simulink model "p1_MCU"  (R2023a)
settings: Solver=FixedStepDiscrete  StartTime=0.0  StopTime=inf  FixedStep=Ts_MCU  RelTol=1e-3  EnableMultiTasking=on
PreLoadFcn:
  | p1_params_new
  | spiDataDefinition
InitFcn:
  | mbd_s32k_consistency_checks(bdroot(gcs));
undefined symbols (not defined in the file or in its folder): ack, cpr_handwheel, cpr_steering, Discrete, DriverInput, DrivetrainLeft, DrivetrainRight, LQFP, MPU_IO, n_handwheel, n_steering, p1data, p1params, param, sr, steering_limit, SteeringLeft, SteeringRight, Time, Ts_MCU, wc, WheelForceLeft, WheelForceRight
libraries: simulink x74, mbd_s32k1xx_ec_toolbox x58, Library_Drivetrain x5, Library_Steering x5, etargetslib x3, ctrlSharedLib x1
(part 3 of 4)

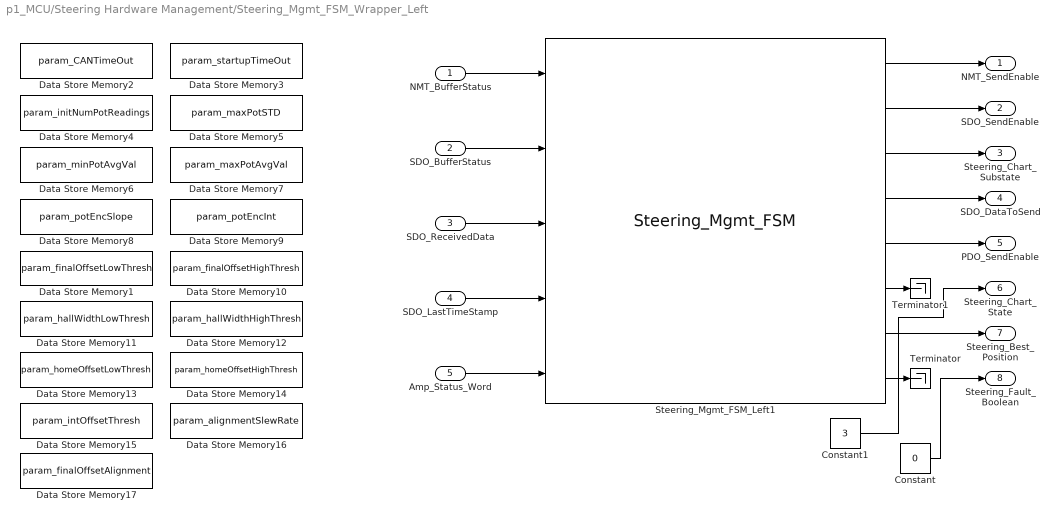
== system p1_MCU/Steering Hardware Management/Steering_Mgmt_FSM_Wrapper_Left ==
  NMT_BufferStatus : Inport
  SDO_BufferStatus : Inport  Port=2
  SDO_ReceivedData : Inport  Port=3
  SDO_LastTimeStamp : Inport  Port=4
  Amp_Status_Word : Inport  Port=5
  Constant : Constant  Value=0  OutDataTypeStr=Inherit: Inherit via back propagation
  Constant1 : Constant  Value=3  OutDataTypeStr=Inherit: Inherit via back propagation
  Data Store Memory1 : DataStoreMemory  DataStoreName=param_finalOffsetLowThresh  ReadBeforeWriteMsg=warning  WriteAfterWriteMsg=warning  WriteAfterReadMsg=warning  InitialValue=p1params.steering.left.finalOffsetLowThresh  ShowAdditionalParam=off  OutDataTypeStr=double
  Data Store Memory10 : DataStoreMemory  DataStoreName=param_finalOffsetHighThresh  ReadBeforeWriteMsg=warning  WriteAfterWriteMsg=warning  WriteAfterReadMsg=warning  InitialValue=p1params.steering.left.finalOffsetHighThresh  ShowAdditionalParam=off  OutDataTypeStr=double
  Data Store Memory11 : DataStoreMemory  DataStoreName=param_hallWidthLowThresh  ReadBeforeWriteMsg=warning  WriteAfterWriteMsg=warning  WriteAfterReadMsg=warning  InitialValue=p1params.steering.left.hallWidthLowThresh  ShowAdditionalParam=off  OutDataTypeStr=double
  Data Store Memory12 : DataStoreMemory  DataStoreName=param_hallWidthHighThresh  ReadBeforeWriteMsg=warning  WriteAfterWriteMsg=warning  WriteAfterReadMsg=warning  InitialValue=p1params.steering.left.hallWidthHighThresh  ShowAdditionalParam=off  OutDataTypeStr=double
  Data Store Memory13 : DataStoreMemory  DataStoreName=param_homeOffsetLowThresh  ReadBeforeWriteMsg=warning  WriteAfterWriteMsg=warning  WriteAfterReadMsg=warning  InitialValue=p1params.steering.left.homeOffsetLowThresh  ShowAdditionalParam=off  OutDataTypeStr=double
  Data Store Memory14 : DataStoreMemory  DataStoreName=param_homeOffsetHighThresh  ReadBeforeWriteMsg=warning  WriteAfterWriteMsg=warning  WriteAfterReadMsg=warning  InitialValue=p1params.steering.left.homeOffsetHighThresh  ShowAdditionalParam=off  OutDataTypeStr=double
  Data Store Memory15 : DataStoreMemory  DataStoreName=param_intOffsetThresh  ReadBeforeWriteMsg=warning  WriteAfterWriteMsg=warning  WriteAfterReadMsg=warning  InitialValue=p1params.steering.left.intOffsetThresh  ShowAdditionalParam=off  OutDataTypeStr=double
  Data Store Memory16 : DataStoreMemory  DataStoreName=param_alignmentSlewRate  ReadBeforeWriteMsg=warning  WriteAfterWriteMsg=warning  WriteAfterReadMsg=warning  InitialValue=p1params.steering.left.alignmentSlewRate  ShowAdditionalParam=off  OutDataTypeStr=double
  Data Store Memory17 : DataStoreMemory  DataStoreName=param_finalOffsetAlignment  ReadBeforeWriteMsg=warning  WriteAfterWriteMsg=warning  WriteAfterReadMsg=warning  InitialValue=p1params.steering.left.finalOffsetAlignment  ShowAdditionalParam=off  OutDataTypeStr=double
  Data Store Memory2 : DataStoreMemory  DataStoreName=param_CANTimeOut  ReadBeforeWriteMsg=warning  WriteAfterWriteMsg=warning  WriteAfterReadMsg=warning  InitialValue=p1params.steering.left.CANTimeOut  ShowAdditionalParam=off  OutDataTypeStr=double
  Data Store Memory3 : DataStoreMemory  DataStoreName=param_startupTimeOut  ReadBeforeWriteMsg=warning  WriteAfterWriteMsg=warning  WriteAfterReadMsg=warning  InitialValue=p1params.steering.left.startupTimeOut  ShowAdditionalParam=off  OutDataTypeStr=double
  Data Store Memory4 : DataStoreMemory  DataStoreName=param_initNumPotReadings  ReadBeforeWriteMsg=warning  WriteAfterWriteMsg=warning  WriteAfterReadMsg=warning  InitialValue=p1params.steering.left.initNumPotReadings  ShowAdditionalParam=off  OutDataTypeStr=double
  Data Store Memory5 : DataStoreMemory  DataStoreName=param_maxPotSTD  ReadBeforeWriteMsg=warning  WriteAfterWriteMsg=warning  WriteAfterReadMsg=warning  InitialValue=p1params.steering.left.maxPotSTD  ShowAdditionalParam=off  OutDataTypeStr=double
  Data Store Memory6 : DataStoreMemory  DataStoreName=param_minPotAvgVal  ReadBeforeWriteMsg=warning  WriteAfterWriteMsg=warning  WriteAfterReadMsg=warning  InitialValue=p1params.steering.left.minPotAvgVal  ShowAdditionalParam=off  OutDataTypeStr=double
  Data Store Memory7 : DataStoreMemory  DataStoreName=param_maxPotAvgVal  ReadBeforeWriteMsg=warning  WriteAfterWriteMsg=warning  WriteAfterReadMsg=warning  InitialValue=p1params.steering.left.maxPotAvgVal  ShowAdditionalParam=off  OutDataTypeStr=double
  Data Store Memory8 : DataStoreMemory  DataStoreName=param_potEncSlope  ReadBeforeWriteMsg=warning  WriteAfterWriteMsg=warning  WriteAfterReadMsg=warning  InitialValue=p1params.steering.left.potEncSlope  ShowAdditionalParam=off  OutDataTypeStr=double
  Data Store Memory9 : DataStoreMemory  DataStoreName=param_potEncInt  ReadBeforeWriteMsg=warning  WriteAfterWriteMsg=warning  WriteAfterReadMsg=warning  InitialValue=p1params.steering.left.potEncInt  ShowAdditionalParam=off  OutDataTypeStr=double
  Steering_Mgmt_FSM_Left1 : Library_Steering/Steering_Mgmt_FSM  SystemSampleTime=-1  VariantActivationTime=update diagram  Latency=0  AutoFrameSizeCalculation=off
  Terminator : Terminator
  Terminator1 : Terminator
  NMT_SendEnable : Outport
  SDO_SendEnable : Outport  Port=2
  Steering_Chart_Substate : Outport  Port=3
  SDO_DataToSend : Outport  Port=4
  PDO_SendEnable : Outport  Port=5
  Steering_Chart_State : Outport  Port=6
  Steering_Best_Position : Outport  Port=7
  Steering_Fault_Boolean : Outport  Port=8
  wires:
  Amp_Status_Word/1 -> Steering_Mgmt_FSM_Left1/5
  Steering_Mgmt_FSM_Left1/2 -> SDO_SendEnable/1
  Steering_Mgmt_FSM_Left1/1 -> NMT_SendEnable/1
  SDO_ReceivedData/1 -> Steering_Mgmt_FSM_Left1/3
  SDO_LastTimeStamp/1 -> Steering_Mgmt_FSM_Left1/4
  SDO_BufferStatus/1 -> Steering_Mgmt_FSM_Left1/2
  NMT_BufferStatus/1 -> Steering_Mgmt_FSM_Left1/1
  Steering_Mgmt_FSM_Left1/8 -> Terminator/1
  Steering_Mgmt_FSM_Left1/7 -> Steering_Best_Position/1
  Steering_Mgmt_FSM_Left1/3 -> Steering_Chart_Substate/1
  Steering_Mgmt_FSM_Left1/4 -> SDO_DataToSend/1
  Steering_Mgmt_FSM_Left1/5 -> PDO_SendEnable/1
  Steering_Mgmt_FSM_Left1/6 -> Terminator1/1
  Constant/1 -> Steering_Fault_Boolean/1
  Constant1/1 -> Steering_Chart_State/1

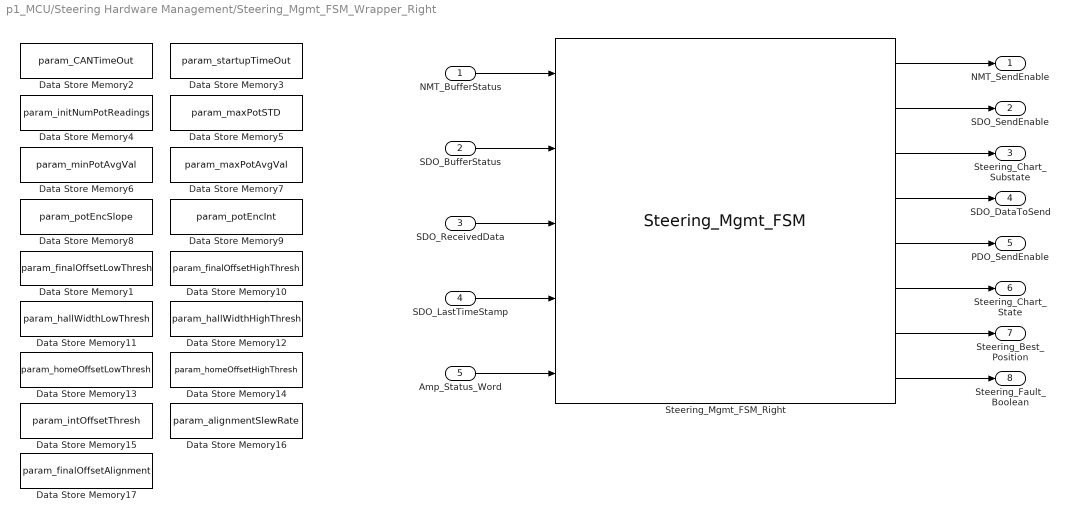
== system p1_MCU/Steering Hardware Management/Steering_Mgmt_FSM_Wrapper_Right ==
  NMT_BufferStatus : Inport
  SDO_BufferStatus : Inport  Port=2
  SDO_ReceivedData : Inport  Port=3
  SDO_LastTimeStamp : Inport  Port=4
  Amp_Status_Word : Inport  Port=5
  Data Store Memory1 : DataStoreMemory  DataStoreName=param_finalOffsetLowThresh  ReadBeforeWriteMsg=warning  WriteAfterWriteMsg=warning  WriteAfterReadMsg=warning  InitialValue=p1params.steering.right.finalOffsetLowThresh  ShowAdditionalParam=off  OutDataTypeStr=double
  Data Store Memory10 : DataStoreMemory  DataStoreName=param_finalOffsetHighThresh  ReadBeforeWriteMsg=warning  WriteAfterWriteMsg=warning  WriteAfterReadMsg=warning  InitialValue=p1params.steering.right.finalOffsetHighThresh  ShowAdditionalParam=off  OutDataTypeStr=double
  Data Store Memory11 : DataStoreMemory  DataStoreName=param_hallWidthLowThresh  ReadBeforeWriteMsg=warning  WriteAfterWriteMsg=warning  WriteAfterReadMsg=warning  InitialValue=p1params.steering.right.hallWidthLowThresh  ShowAdditionalParam=off  OutDataTypeStr=double
  Data Store Memory12 : DataStoreMemory  DataStoreName=param_hallWidthHighThresh  ReadBeforeWriteMsg=warning  WriteAfterWriteMsg=warning  WriteAfterReadMsg=warning  InitialValue=p1params.steering.right.hallWidthHighThresh  ShowAdditionalParam=off  OutDataTypeStr=double
  Data Store Memory13 : DataStoreMemory  DataStoreName=param_homeOffsetLowThresh  ReadBeforeWriteMsg=warning  WriteAfterWriteMsg=warning  WriteAfterReadMsg=warning  InitialValue=p1params.steering.right.homeOffsetLowThresh  ShowAdditionalParam=off  OutDataTypeStr=double
  Data Store Memory14 : DataStoreMemory  DataStoreName=param_homeOffsetHighThresh  ReadBeforeWriteMsg=warning  WriteAfterWriteMsg=warning  WriteAfterReadMsg=warning  InitialValue=p1params.steering.right.homeOffsetHighThresh  ShowAdditionalParam=off  OutDataTypeStr=double
  Data Store Memory15 : DataStoreMemory  DataStoreName=param_intOffsetThresh  ReadBeforeWriteMsg=warning  WriteAfterWriteMsg=warning  WriteAfterReadMsg=warning  InitialValue=p1params.steering.right.intOffsetThresh  ShowAdditionalParam=off  OutDataTypeStr=double
  Data Store Memory16 : DataStoreMemory  DataStoreName=param_alignmentSlewRate  ReadBeforeWriteMsg=warning  WriteAfterWriteMsg=warning  WriteAfterReadMsg=warning  InitialValue=p1params.steering.right.alignmentSlewRate  ShowAdditionalParam=off  OutDataTypeStr=double
  Data Store Memory17 : DataStoreMemory  DataStoreName=param_finalOffsetAlignment  ReadBeforeWriteMsg=warning  WriteAfterWriteMsg=warning  WriteAfterReadMsg=warning  InitialValue=p1params.steering.right.finalOffsetAlignment  ShowAdditionalParam=off  OutDataTypeStr=double
  Data Store Memory2 : DataStoreMemory  DataStoreName=param_CANTimeOut  ReadBeforeWriteMsg=warning  WriteAfterWriteMsg=warning  WriteAfterReadMsg=warning  InitialValue=p1params.steering.right.CANTimeOut  ShowAdditionalParam=off  OutDataTypeStr=double
  Data Store Memory3 : DataStoreMemory  DataStoreName=param_startupTimeOut  ReadBeforeWriteMsg=warning  WriteAfterWriteMsg=warning  WriteAfterReadMsg=warning  InitialValue=p1params.steering.right.startupTimeOut  ShowAdditionalParam=off  OutDataTypeStr=double
  Data Store Memory4 : DataStoreMemory  DataStoreName=param_initNumPotReadings  ReadBeforeWriteMsg=warning  WriteAfterWriteMsg=warning  WriteAfterReadMsg=warning  InitialValue=p1params.steering.right.initNumPotReadings  ShowAdditionalParam=off  OutDataTypeStr=double
  Data Store Memory5 : DataStoreMemory  DataStoreName=param_maxPotSTD  ReadBeforeWriteMsg=warning  WriteAfterWriteMsg=warning  WriteAfterReadMsg=warning  InitialValue=p1params.steering.right.maxPotSTD  ShowAdditionalParam=off  OutDataTypeStr=double
  Data Store Memory6 : DataStoreMemory  DataStoreName=param_minPotAvgVal  ReadBeforeWriteMsg=warning  WriteAfterWriteMsg=warning  WriteAfterReadMsg=warning  InitialValue=p1params.steering.right.minPotAvgVal  ShowAdditionalParam=off  OutDataTypeStr=double
  Data Store Memory7 : DataStoreMemory  DataStoreName=param_maxPotAvgVal  ReadBeforeWriteMsg=warning  WriteAfterWriteMsg=warning  WriteAfterReadMsg=warning  InitialValue=p1params.steering.right.maxPotAvgVal  ShowAdditionalParam=off  OutDataTypeStr=double
  Data Store Memory8 : DataStoreMemory  DataStoreName=param_potEncSlope  ReadBeforeWriteMsg=warning  WriteAfterWriteMsg=warning  WriteAfterReadMsg=warning  InitialValue=p1params.steering.right.potEncSlope  ShowAdditionalParam=off  OutDataTypeStr=double
  Data Store Memory9 : DataStoreMemory  DataStoreName=param_potEncInt  ReadBeforeWriteMsg=warning  WriteAfterWriteMsg=warning  WriteAfterReadMsg=warning  InitialValue=p1params.steering.right.potEncInt  ShowAdditionalParam=off  OutDataTypeStr=double
  Steering_Mgmt_FSM_Right : Library_Steering/Steering_Mgmt_FSM  SystemSampleTime=-1  VariantActivationTime=update diagram  Latency=0  AutoFrameSizeCalculation=off
  NMT_SendEnable : Outport
  SDO_SendEnable : Outport  Port=2
  Steering_Chart_Substate : Outport  Port=3
  SDO_DataToSend : Outport  Port=4
  PDO_SendEnable : Outport  Port=5
  Steering_Chart_State : Outport  Port=6
  Steering_Best_Position : Outport  Port=7
  Steering_Fault_Boolean : Outport  Port=8
  wires:
  Amp_Status_Word/1 -> Steering_Mgmt_FSM_Right/5
  Steering_Mgmt_FSM_Right/2 -> SDO_SendEnable/1
  Steering_Mgmt_FSM_Right/1 -> NMT_SendEnable/1
  SDO_ReceivedData/1 -> Steering_Mgmt_FSM_Right/3
  SDO_LastTimeStamp/1 -> Steering_Mgmt_FSM_Right/4
  SDO_BufferStatus/1 -> Steering_Mgmt_FSM_Right/2
  NMT_BufferStatus/1 -> Steering_Mgmt_FSM_Right/1
  Steering_Mgmt_FSM_Right/8 -> Steering_Fault_Boolean/1
  Steering_Mgmt_FSM_Right/7 -> Steering_Best_Position/1
  Steering_Mgmt_FSM_Right/3 -> Steering_Chart_Substate/1
  Steering_Mgmt_FSM_Right/4 -> SDO_DataToSend/1
  Steering_Mgmt_FSM_Right/5 -> PDO_SendEnable/1
  Steering_Mgmt_FSM_Right/6 -> Steering_Chart_State/1

== system p1_MCU/Subsystem/System Start ==

== system p1_MCU/Subsystem1/piSPISend ==
  Data Store Memory1 : DataStoreMemory  DataStoreName=spiTx  ReadBeforeWriteMsg=warning  WriteAfterWriteMsg=warning  WriteAfterReadMsg=warning  InitialValue=zeros(p1data.spiBytes,1)  ShowAdditionalParam=off  OutDataTypeStr=uint8
  Data Store Memory3 : DataStoreMemory  DataStoreName=spiPadding  ReadBeforeWriteMsg=warning  WriteAfterWriteMsg=warning  WriteAfterReadMsg=warning  InitialValue=zeros(p1data.mcuPadding,1)  ShowAdditionalParam=off  OutDataTypeStr=uint8
  Data Store Read1 : DataStoreRead  DataStoreName=spiTx  IndexOptions=Index vector (dialog)  Indices=1  OutputSizes=1
  Data Store Read10 : DataStoreRead  DataStoreName=WheelForceRight  IndexOptions=Index vector (dialog)  Indices=1  OutputSizes=1
  Data Store Read11 : DataStoreRead  DataStoreName=spiRx  IndexOptions=Index vector (dialog)  Indices=1  OutputSizes=1
  Data Store Read12 : DataStoreRead  DataStoreName=IMU  IndexOptions=Index vector (dialog)  Indices=1  OutputSizes=1
  Data Store Read14 : DataStoreRead  DataStoreName=spiPadding  IndexOptions=Index vector (dialog)  Indices=1  OutputSizes=1
  Data Store Read2 : DataStoreRead  DataStoreName=IgnState  IndexOptions=Index vector (dialog)  Indices=1  OutputSizes=1
  Data Store Read3 : DataStoreRead  DataStoreName=ControlPanel  IndexOptions=Index vector (dialog)  Indices=1  OutputSizes=1
  Data Store Read4 : DataStoreRead  DataStoreName=SteeringRight  IndexOptions=Index vector (dialog)  Indices=1  OutputSizes=1
  Data Store Read5 : DataStoreRead  DataStoreName=DriverInput  IndexOptions=Index vector (dialog)  Indices=1  OutputSizes=1
  Data Store Read6 : DataStoreRead  DataStoreName=SteeringLeft  IndexOptions=Index vector (dialog)  Indices=1  OutputSizes=1
  Data Store Read7 : DataStoreRead  DataStoreName=DrivetrainLeft  IndexOptions=Index vector (dialog)  Indices=1  OutputSizes=1
  Data Store Read8 : DataStoreRead  DataStoreName=DrivetrainRight  IndexOptions=Index vector (dialog)  Indices=1  OutputSizes=1
  Data Store Read9 : DataStoreRead  DataStoreName=WheelForceLeft  IndexOptions=Index vector (dialog)  Indices=1  OutputSizes=1
  Data Store Write1 : DataStoreWrite  DataStoreName=spiTx  IndexOptions=Index vector (dialog)  Indices=1  OutputSizes=1
  Data Store Write2 : DataStoreWrite  DataStoreName=spiRx  IndexOptions=Index vector (dialog)  Indices=1  OutputSizes=1
  Data Store Write3 : DataStoreWrite  DataStoreName=MPU_IO  IndexOptions=Index vector (dialog)  Indices=1  OutputSizes=1
  Data Store Write5 : DataStoreWrite  DataStoreName=GPS  IndexOptions=Index vector (dialog)  Indices=1  OutputSizes=1
  Demux : Demux  Outputs=3
  Footer : Constant  Value=[0 0 101 110 100]  OutDataTypeStr=uint8
  Header : Constant  Value=[115 116 97 114 116 0 0 0 0 0]  OutDataTypeStr=uint8
  LPSPI_Slave_Transfer : mbd_s32k1xx_ec_toolbox/Communication Blocks/SPI Blocks/LPSPI_Slave_Transfer  instance=1  pcs=3  pcs_polarity=ActiveLow  xfermode=Non blocking  timeout=70  spi_upd=on
  Mux1 : Mux  Inputs=13
  Terminator : Terminator
  wires:
  Data Store Read8/1 -> Mux1/8
  Data Store Read2/1 -> Mux1/2
  Data Store Read4/1 -> Mux1/6
  Mux1/1 -> Data Store Write1/1
  LPSPI_Slave_Transfer/1 -> Data Store Write2/1
  Data Store Read1/1 -> LPSPI_Slave_Transfer/1
  Data Store Read11/1 -> Demux/1
  Data Store Read6/1 -> Mux1/5
  Data Store Read7/1 -> Mux1/7
  Data Store Read5/1 -> Mux1/4
  Data Store Read3/1 -> Mux1/3
  Demux/3 -> Terminator/1
  Demux/1 -> Data Store Write5/1
  Demux/2 -> Data Store Write3/1
  Data Store Read10/1 -> Mux1/11
  Data Store Read9/1 -> Mux1/10
  Data Store Read12/1 -> Mux1/9
  Header/1 -> Mux1/1
  Data Store Read14/1 -> Mux1/12
  Footer/1 -> Mux1/13

== system p1_MCU/Subsystem2/If Action Subsystem ==
  note: Start interrupt-based reception
      | on CAN1 bus
  note: Enable CAN1 bus
  note: Hold Power On (Ignition)
  note: Enable 5V Output
  note: Enable CAN0 bus
  note: Start interrupt-based reception
      | on CAN0 bus
  note: Enable CAN2 bus
  note: Enable Digital Outputs
  note: Enable Digital Input Pullups
  Action Port : ActionPort  ActionPortLabel=if(u1 == 0)
  Constant : Constant  OutDataTypeStr=uint32
  Constant{1..2,5..6} (4 alike) : Constant  OutDataTypeStr=Inherit: Inherit via back propagation
  Constant3 : Constant  Value=0  OutDataTypeStr=Inherit: Inherit via back propagation
  Constant4 : Constant  Value=0  OutDataTypeStr=Inherit: Inherit via back propagation
  Constant9 : Constant  Value=0  OutDataTypeStr=Inherit: Inherit via back propagation
  Digital_Output : mbd_s32k1xx_ec_toolbox/GPIO Blocks/Digital_Output  gpio_pin=PTA14: [PTA14 | Port A I/O]  init_val=Low  drive_strength=Low
  Digital_Output1 : mbd_s32k1xx_ec_toolbox/GPIO Blocks/Digital_Output  gpio_pin=PTE7: [PTE7 | Port E I/O]  init_val=Low  drive_strength=Low
  Digital_Output2 : mbd_s32k1xx_ec_toolbox/GPIO Blocks/Digital_Output  gpio_pin=PTD7: [PTD7 | Port D I/O]  init_val=High  drive_strength=Low
  Digital_Output3 : mbd_s32k1xx_ec_toolbox/GPIO Blocks/Digital_Output  gpio_pin=PTC10: [PTC10 | Port C I/O]  init_val=Low  drive_strength=Low
  Digital_Output4 : mbd_s32k1xx_ec_toolbox/GPIO Blocks/Digital_Output  gpio_pin=PTD6: [PTD6 | Port D I/O]  init_val=Low  drive_strength=Low
  Digital_Output5 : mbd_s32k1xx_ec_toolbox/GPIO Blocks/Digital_Output  gpio_pin=PTE3: [PTE3 | Port E I/O]  init_val=Low  drive_strength=Low
  Digital_Output6 : mbd_s32k1xx_ec_toolbox/GPIO Blocks/Digital_Output  gpio_pin=PTC8: [PTC8 | Port C I/O]  init_val=Low  drive_strength=Low
  Enable_Handwheel_Index_Capture_Once : mbd_s32k1xx_ec_toolbox/GPIO Blocks/Digital_Input_ISR_Enable_Disable  gpio_pin=PTD10: [PTD10 | Port D I/O]  irqc=on either-edge
  FCAN_Receive : mbd_s32k1xx_ec_toolbox/Communication Blocks/CAN Blocks/FCAN_Receive  can_instance=1  can_mode=Non-blocking  can_timeout_ms=0  can_mb_idx=0  can_extended_id=off  can_is_remote=off  can_id=0  can_msg_mask=0  show_adv_opts=off  can_use_rxfifo=off  can_fd_enable=off
  FCAN_Receive1 : mbd_s32k1xx_ec_toolbox/Communication Blocks/CAN Blocks/FCAN_Receive  can_instance=0  can_mode=Non-blocking  can_timeout_ms=0  can_mb_idx=0  can_extended_id=off  can_is_remote=off  can_id=0  can_msg_mask=0  show_adv_opts=off  can_use_rxfifo=off  can_fd_enable=off
  FCAN_Receive2 : mbd_s32k1xx_ec_toolbox/Communication Blocks/CAN Blocks/FCAN_Receive  can_instance=2  can_mode=Non-blocking  can_timeout_ms=0  can_mb_idx=7  can_extended_id=off  can_is_remote=off  can_id=0  can_msg_mask=0  show_adv_opts=off  can_use_rxfifo=off  can_fd_enable=off
  IMU Reception : Subsystem
  Init Flag Write : DataStoreWrite  DataStoreName=init_flag  IndexOptions=Index vector (dialog)  Indices=1  OutputSizes=1
  wires:
  Constant/1 -> Init Flag Write/1
  Constant9/1 -> Digital_Output/1
  Constant2/1 -> Digital_Output2/1
  Constant1/1 -> Digital_Output1/1
  Constant3/1 -> Digital_Output3/1
  Constant4/1 -> Digital_Output4/1
  Constant5/1 -> Digital_Output5/1
  Constant6/1 -> Digital_Output6/1

== system p1_MCU/WFT CAN Receive/Function-Call Subsystem ==
  Message Buffer : Inport
  MSG ID : Inport  Port=2
  Data Packet : Inport  Port=3
  Data Length : Inport  Port=4
  Time Stamp : Inport  Port=5
  function : TriggerPort  TriggerType=function-call  VariantControl=Variant
  Accurate Feedback2 : Subsystem  TreatAsAtomicUnit=on
      settings: RTWSystemCode=Inline
  Accurate Feedback3 : Subsystem  TreatAsAtomicUnit=on
      settings: RTWSystemCode=Inline
  Bus Creator : BusCreator  Inputs=10
  Bus Creator1 : BusCreator  Inputs=10
  Data Store Write1 : DataStoreWrite  DataStoreName=WheelForceLeft  DataStoreElements=WheelForceLeft(1:8)  IndexOptions=Index vector (dialog)  Indices=1  OutputSizes=1
  Data Store Write2 : DataStoreWrite  DataStoreName=WheelForceLeft  DataStoreElements=WheelForceLeft(9:16)  IndexOptions=Index vector (dialog)  Indices=1  OutputSizes=1
  Data Store Write3 : DataStoreWrite  DataStoreName=WheelForceRight  DataStoreElements=WheelForceRight(1:8)  IndexOptions=Index vector (dialog)  Indices=1  OutputSizes=1
  Data Store Write4 : DataStoreWrite  DataStoreName=WheelForceRight  DataStoreElements=WheelForceRight(9:16)  IndexOptions=Index vector (dialog)  Indices=1  OutputSizes=1
  Data Store Write5 : DataStoreWrite  DataStoreName=WheelForceLeft  DataStoreElements=WheelForceLeft(17:20)  IndexOptions=Index vector (dialog)  Indices=1  OutputSizes=1
  Data Store Write6 : DataStoreWrite  DataStoreName=WheelForceRight  DataStoreElements=WheelForceRight(17:20)  IndexOptions=Index vector (dialog)  Indices=1  OutputSizes=1
  FCAN_Receive : mbd_s32k1xx_ec_toolbox/Communication Blocks/CAN Blocks/FCAN_Receive  can_instance=2  can_mode=Non-blocking  can_timeout_ms=0  can_mb_idx=7  can_extended_id=off  can_is_remote=off  can_id=0  can_msg_mask=0  show_adv_opts=off  can_use_rxfifo=off  can_fd_enable=off
  Switch Case : SwitchCase  CaseConditions={hex2dec('1CC'),hex2dec('5CC'),hex2dec('3CC'),hex2dec('1C7'),hex2dec('5C7'),hex2dec('3C7')}  ShowDefaultCase=off
  Terminator : Terminator
  Terminator1 : Terminator
  Terminator2 : Terminator
  WFT Packet 1 Left : Subsystem  TreatAsAtomicUnit=on
      settings: RTWSystemCode=Inline
  WFT Packet 1 Left1 : Subsystem  TreatAsAtomicUnit=on
      settings: RTWSystemCode=Inline
  WFT Packet 1 Left2 : Subsystem  TreatAsAtomicUnit=on
      settings: RTWSystemCode=Inline
  WFT Packet 1 Left3 : Subsystem  TreatAsAtomicUnit=on
      settings: RTWSystemCode=Inline
  WFT Feedback Left : Outport
  WFT Feedback Right : Outport  Port=2
  wires:
  WFT Packet 1 Left/2(Fx) -> Bus Creator/1  "Fx Left"
  WFT Packet 1 Left/1(Save Data) -> Data Store Write1/1
  WFT Packet 1 Left/4(Fz) -> Bus Creator/3  "Fz Left"
  Switch Case/1 -> WFT Packet 1 Left/Action
  WFT Packet 1 Left/5(Mx) -> Bus Creator/4  "Mx Left"
  Data Length/1 -> Terminator/1
  Bus Creator/1 -> WFT Feedback Left/1
  Message Buffer/1 -> Terminator1/1
  MSG ID/1 -> Switch Case/1
  WFT Packet 1 Left/3(Fy) -> Bus Creator/2  "Fy Left"
  Data Packet/1 -> WFT Packet 1 Left3/1(Data Packet), Accurate Feedback3/1(Data Packet), Accurate Feedback2/1(Data Packet), WFT Packet 1 Left2/1(Data Packet), WFT Packet 1 Left1/1(Data Packet), WFT Packet 1 Left/1(Data Packet)
  WFT Packet 1 Left1/1(Save Data) -> Data Store Write2/1
  WFT Packet 1 Left1/5(Pos) -> Bus Creator/8  "Pos Left"
  WFT Packet 1 Left1/3(Mz) -> Bus Creator/6  "Mz Left"
  WFT Packet 1 Left1/4(Vel) -> Bus Creator/7  "Vel Left"
  Switch Case/2 -> WFT Packet 1 Left1/Action
  WFT Packet 1 Left1/2(My) -> Bus Creator/5  "My Left"
  Accurate Feedback2/1(Save Data) -> Data Store Write3/1
  Switch Case/5 -> Accurate Feedback3/Action
  Accurate Feedback3/1(Save Data) -> Data Store Write4/1
  Switch Case/4 -> Accurate Feedback2/Action
  WFT Packet 1 Left2/2(Ax) -> Bus Creator/9  "Ax Left"
  Switch Case/3 -> WFT Packet 1 Left2/Action
  WFT Packet 1 Left2/3(Az) -> Bus Creator/10  "Ay Left"
  WFT Packet 1 Left2/1(Save Data) -> Data Store Write5/1
  Switch Case/6 -> WFT Packet 1 Left3/Action
  Accurate Feedback3/4(Vel) -> Bus Creator1/7  "Vel Right"
  Accurate Feedback3/2(My) -> Bus Creator1/5  "My Right"
  Accurate Feedback2/5(Mx) -> Bus Creator1/4  "Mx Right"
  Accurate Feedback2/3(Fy) -> Bus Creator1/2  "Fy Right"
  WFT Packet 1 Left3/3(Az) -> Bus Creator1/10  "Ay Right"
  Bus Creator1/1 -> WFT Feedback Right/1
  Accurate Feedback2/2(Fx) -> Bus Creator1/1  "Fx Right"
  WFT Packet 1 Left3/2(Ax) -> Bus Creator1/9  "Ax Right"
  Accurate Feedback3/3(Mz) -> Bus Creator1/6  "Mz Right"
  Accurate Feedback3/5(Pos) -> Bus Creator1/8  "Pos Right"
  Accurate Feedback2/4(Fz) -> Bus Creator1/3  "Fz Right"
  WFT Packet 1 Left3/1(Save Data) -> Data Store Write6/1
  Time Stamp/1 -> Terminator2/1

== system p1_MCU/ Controls Data Reception/Function-Call Subsystem1/If Action Subsystem ==
  Raw Encoder Estimate : Inport
  Fused Angle Estimate : Inport  Port=2
  SimTime : Inport  Port=3
  Action Port : ActionPort  ActionPortLabel=if(u1 > 0.1)
  1-D Lookup Table : Lookup_n-D  NumberOfTableDimensions=1  BreakpointsForDimension1=pi/180*[-7.2*30:7.2:30*7.2]  Table=pi/180*[-7.2*30:7.2:30*7.2]  InterpMethod=Nearest  InternalRulePriority=Speed  RndMeth=Simplest
  Digital_Input_ISR_Enable_Disable : mbd_s32k1xx_ec_toolbox/GPIO Blocks/Digital_Input_ISR_Enable_Disable  gpio_pin=PTD10: [PTD10 | Port D I/O]  irqc=request disabled
  Subtract : Sum  Inputs=-+
  Latched Encoder Offset : Outport  InitialOutput=[0]
  Time of Latch : Outport  Port=2  InitialOutput=[0]
  wires:
  Subtract/1 -> Latched Encoder Offset/1
  Fused Angle Estimate/1 -> 1-D Lookup Table/1
  Raw Encoder Estimate/1 -> Subtract/2
  1-D Lookup Table/1 -> Subtract/1
  SimTime/1 -> Time of Latch/1

== system p1_MCU/Steering Control/Steering Controller/Ackermann Correction ==
  Ackermann Angle : Inport
  left ackermann ideal correction angle : Fcn  Expr=u/(1-u*ack*param.d/2/(param.a+param.b))
  right ackermann ideal correction angle : Fcn  Expr=u/(1+u*ack*param.d/2/(param.a+param.b))
  L Steer Angle : Outport
  R Steer Angle : Outport  Port=2
  wires:
  Ackermann Angle/1 -> right ackermann ideal correction angle/1, left ackermann ideal correction angle/1
  right ackermann ideal correction angle/1 -> R Steer Angle/1
  left ackermann ideal correction angle/1 -> L Steer Angle/1

== system p1_MCU/Steering Control/Steering Controller/HAL-9000 ==
  Trigger : Inport
  Amplitude : Constant  Value=amplitude*sr*pi/180
  Chirp Signal : Subsystem  mask(chirp){f1=startfreq, T=duration, f2=endfreq, VectorParams1D=on}
      mask prompts: f1 "Initial frequency (Hz):"; T "Target time (secs):"; f2 "Frequency at target time (Hz):"; VectorParams1D "Interpret vectors parameters as 1-D"
      mask help: Output a linear chirp signal (sine wave whose frequency varies linearly with time).
      mask init:
      | blkName = gcb;
      | t=[0:.1:5];
      | set_param([blkName '/targetTime'], 'VectorParams1D', VectorParams1D);
      | set_param([blkName '/initialFreq'], 'VectorParams1D', VectorParams1D);
      | set_param([blkName '/deltaFreq'], 'VectorParams1D', VectorParams1D);
      mask Help: The chirp signal has linearly increasing frequency with time.  This block can be used for spectral analysis of nonlinear systems.
      mask Display: plot(t,sin(t.*t))
  Constant : Constant
  Constant1 : Constant  Value=0
  Delay : Constant  Value=delay
  Digital Clock : DigitalClock  SampleTime=Ts_MCU
  Double chirp : Subsystem
  Double-step : Subsystem
      mask Display: plot([0 1 1 2 2 3 3 4 4 5],[0 0 1 1 0 0 -1 -1 0 0])
  Enable : Constant  Value=enabled
  Latch : Subsystem  TreatAsAtomicUnit=on
  Maneuver : Constant  Value=maneuver
  Multiport Switch : MultiPortSwitch  Inputs=5  SaturateOnIntegerOverflow=off  InputSameDT=off
  Product : Product  Inputs=3  SaturateOnIntegerOverflow=on  OutDataTypeStr=Inherit: Same as first input
  Product1 : Product  SaturateOnIntegerOverflow=on  OutDataTypeStr=Inherit: Same as first input
  Ramp : Subsystem
      mask Display: plot([0 3 7 10],[1 1 8 8])
  Step : Subsystem
      mask Display: plot([0 5 5 10],[1 1 8 8])
  Sum : Sum  Inputs=|++
  Switch : Switch  Criteria=u2 ~= 0  SaturateOnIntegerOverflow=off  InputSameDT=off
  Offset : Outport
  wires:
  Double chirp/1(Out1) -> Multiport Switch/6
  Double-step/1(Out) -> Multiport Switch/5
  Enable/1 -> Product1/2
  Trigger/1 -> Switch/2
  Delay/1 -> Sum/2
  Latch/1(Out1) -> Sum/1
  Chirp Signal/1(Out2) -> Multiport Switch/4
  Ramp/1(Out1) -> Multiport Switch/3
  Sum/1 -> Double chirp/1(In1), Double-step/1(Start Time), Chirp Signal/1(Start Time), Ramp/1(Start Time), Step/1(Start Time)
  Maneuver/1 -> Multiport Switch/1
  Step/1(Out) -> Multiport Switch/2
  Amplitude/1 -> Product/3
  Multiport Switch/1 -> Product/2
  Product/1 -> Offset/1
  Product1/1 -> Latch/Trigger, Product/1
  Digital Clock/1 -> Latch/1(In1)
  Switch/1 -> Product1/1
  Constant1/1 -> Switch/3
  Constant/1 -> Switch/1

== system p1_MCU/Subsystem2/If Action Subsystem/IMU Reception ==
  Constant1 : Constant  Value=[hex2dec('10'); hex2dec('50'); hex2dec('50')]  OutDataTypeStr=uint8
  LPSPI_Master_Transfer : mbd_s32k1xx_ec_toolbox/Communication Blocks/SPI Blocks/LPSPI_Master_Transfer  instance=0  pcs=2  pcs_polarity=ActiveLow  xfermode=Non blocking  timeout=50  spi_upd=on
  Terminator : Terminator
  wires:
  Constant1/1 -> LPSPI_Master_Transfer/1
  LPSPI_Master_Transfer/1 -> Terminator/1

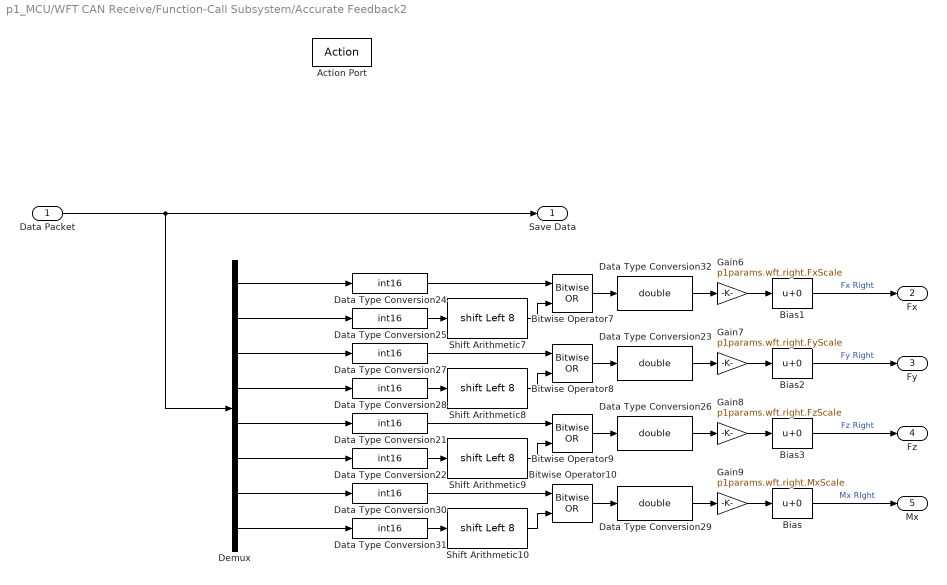
== system p1_MCU/WFT CAN Receive/Function-Call Subsystem/Accurate Feedback2 ==
  Data Packet : Inport
  Action Port : ActionPort  ActionPortLabel=case [ 455 ]:
  Bias{,1..3} (4 alike) : Bias  SaturateOnIntegerOverflow=off
  Bitwise Operator{7..10} (4 alike) : simulink/Logic and Bit Operations/Bitwise Operator  logicop=OR  UseBitMask=off  NumInputPorts=2  BitMask=bin2dec('11011001')  BitMaskRealWorld=Stored Integer
  Data Type Conversion{21..22,24..25,27..28,30..31} (8 alike) : DataTypeConversion  OutDataTypeStr=int16  SaturateOnIntegerOverflow=off  RndMeth=Floor
  Data Type Conversion{23,26,29,32} (4 alike) : DataTypeConversion  OutDataTypeStr=double  SaturateOnIntegerOverflow=off  RndMeth=Floor
  Demux : Demux  Outputs=8
  Gain6 : Gain  Gain=p1params.wft.right.FxScale  OutDataTypeStr=Inherit: Inherit via back propagation
  Gain7 : Gain  Gain=p1params.wft.right.FyScale  OutDataTypeStr=Inherit: Inherit via back propagation
  Gain8 : Gain  Gain=p1params.wft.right.FzScale  OutDataTypeStr=Inherit: Inherit via back propagation
  Gain9 : Gain  Gain=p1params.wft.right.MxScale  OutDataTypeStr=Inherit: Inherit via back propagation
  Shift Arithmetic{7..10} (4 alike) : ArithShift  BitShiftNumber=8  BitShiftDirection=Left
  Save Data : Outport
  Fx : Outport  Port=2
  Fy : Outport  Port=3
  Fz : Outport  Port=4
  Mx : Outport  Port=5
  wires:
  Data Packet/1 -> Save Data/1, Demux/1
  Demux/8 -> Data Type Conversion31/1
  Demux/7 -> Data Type Conversion30/1
  Demux/6 -> Data Type Conversion22/1
  Demux/5 -> Data Type Conversion21/1
  Demux/4 -> Data Type Conversion28/1
  Demux/3 -> Data Type Conversion27/1
  Demux/2 -> Data Type Conversion25/1
  Demux/1 -> Data Type Conversion24/1
  Data Type Conversion23/1 -> Gain7/1
  Shift Arithmetic9/1 -> Bitwise Operator9/2
  Shift Arithmetic8/1 -> Bitwise Operator8/2
  Data Type Conversion25/1 -> Shift Arithmetic7/1
  Data Type Conversion31/1 -> Shift Arithmetic10/1
  Bitwise Operator7/1 -> Data Type Conversion32/1
  Data Type Conversion29/1 -> Gain9/1
  Data Type Conversion27/1 -> Bitwise Operator8/1
  Shift Arithmetic10/1 -> Bitwise Operator10/2
  Gain6/1 -> Bias1/1
  Bitwise Operator8/1 -> Data Type Conversion23/1
  Bitwise Operator10/1 -> Data Type Conversion29/1
  Data Type Conversion26/1 -> Gain8/1
  Gain8/1 -> Bias3/1
  Shift Arithmetic7/1 -> Bitwise Operator7/2
  Data Type Conversion32/1 -> Gain6/1
  Data Type Conversion28/1 -> Shift Arithmetic8/1
  Gain9/1 -> Bias/1
  Bitwise Operator9/1 -> Data Type Conversion26/1
  Data Type Conversion21/1 -> Bitwise Operator9/1
  Data Type Conversion22/1 -> Shift Arithmetic9/1
  Data Type Conversion30/1 -> Bitwise Operator10/1
  Gain7/1 -> Bias2/1
  Data Type Conversion24/1 -> Bitwise Operator7/1
  Bias/1 -> Mx/1  "Mx RIght"
  Bias3/1 -> Fz/1  "Fz Right"
  Bias2/1 -> Fy/1  "Fy Right"
  Bias1/1 -> Fx/1  "Fx Right"

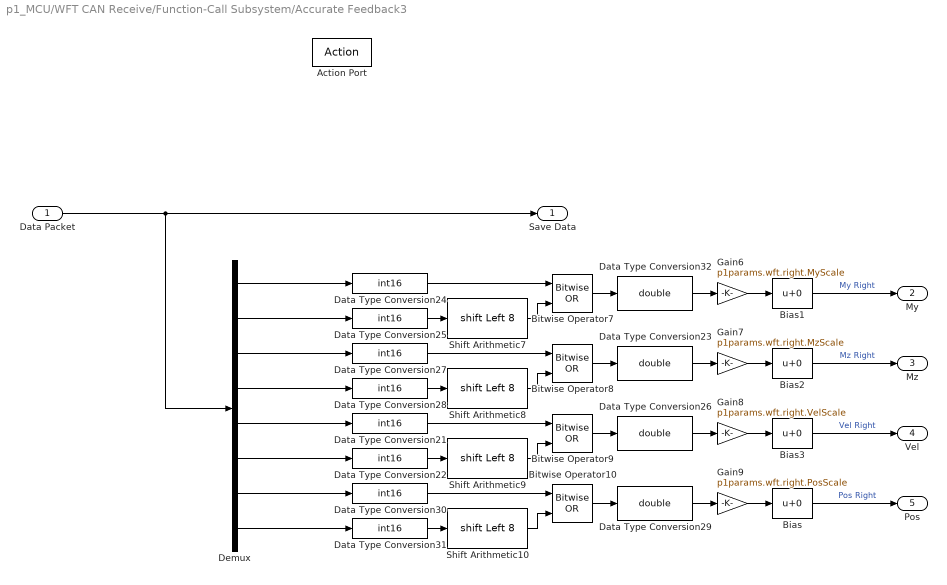
== system p1_MCU/WFT CAN Receive/Function-Call Subsystem/Accurate Feedback3 ==
  Data Packet : Inport
  Action Port : ActionPort  ActionPortLabel=case [ 1479 ]:
  Bias{,1..3} (4 alike) : Bias  SaturateOnIntegerOverflow=off
  Bitwise Operator{7..10} (4 alike) : simulink/Logic and Bit Operations/Bitwise Operator  logicop=OR  UseBitMask=off  NumInputPorts=2  BitMask=bin2dec('11011001')  BitMaskRealWorld=Stored Integer
  Data Type Conversion{21..22,24..25,27..28,30..31} (8 alike) : DataTypeConversion  OutDataTypeStr=int16  SaturateOnIntegerOverflow=off  RndMeth=Floor
  Data Type Conversion{23,26,29,32} (4 alike) : DataTypeConversion  OutDataTypeStr=double  SaturateOnIntegerOverflow=off  RndMeth=Floor
  Demux : Demux  Outputs=8
  Gain6 : Gain  Gain=p1params.wft.right.MyScale  OutDataTypeStr=Inherit: Inherit via back propagation
  Gain7 : Gain  Gain=p1params.wft.right.MzScale  OutDataTypeStr=Inherit: Inherit via back propagation
  Gain8 : Gain  Gain=p1params.wft.right.VelScale  OutDataTypeStr=Inherit: Inherit via back propagation
  Gain9 : Gain  Gain=p1params.wft.right.PosScale  OutDataTypeStr=Inherit: Inherit via back propagation
  Shift Arithmetic{7..10} (4 alike) : ArithShift  BitShiftNumber=8  BitShiftDirection=Left
  Save Data : Outport
  My : Outport  Port=2
  Mz : Outport  Port=3
  Vel : Outport  Port=4
  Pos : Outport  Port=5
  wires:
  Data Packet/1 -> Save Data/1, Demux/1
  Demux/8 -> Data Type Conversion31/1
  Demux/7 -> Data Type Conversion30/1
  Demux/6 -> Data Type Conversion22/1
  Demux/5 -> Data Type Conversion21/1
  Demux/4 -> Data Type Conversion28/1
  Demux/3 -> Data Type Conversion27/1
  Demux/2 -> Data Type Conversion25/1
  Demux/1 -> Data Type Conversion24/1
  Data Type Conversion23/1 -> Gain7/1
  Shift Arithmetic9/1 -> Bitwise Operator9/2
  Shift Arithmetic8/1 -> Bitwise Operator8/2
  Data Type Conversion25/1 -> Shift Arithmetic7/1
  Data Type Conversion31/1 -> Shift Arithmetic10/1
  Bitwise Operator7/1 -> Data Type Conversion32/1
  Data Type Conversion29/1 -> Gain9/1
  Data Type Conversion27/1 -> Bitwise Operator8/1
  Shift Arithmetic10/1 -> Bitwise Operator10/2
  Gain6/1 -> Bias1/1
  Bitwise Operator8/1 -> Data Type Conversion23/1
  Bitwise Operator10/1 -> Data Type Conversion29/1
  Data Type Conversion26/1 -> Gain8/1
  Gain8/1 -> Bias3/1
  Shift Arithmetic7/1 -> Bitwise Operator7/2
  Data Type Conversion32/1 -> Gain6/1
  Data Type Conversion28/1 -> Shift Arithmetic8/1
  Gain9/1 -> Bias/1
  Bitwise Operator9/1 -> Data Type Conversion26/1
  Data Type Conversion21/1 -> Bitwise Operator9/1
  Data Type Conversion22/1 -> Shift Arithmetic9/1
  Data Type Conversion30/1 -> Bitwise Operator10/1
  Gain7/1 -> Bias2/1
  Data Type Conversion24/1 -> Bitwise Operator7/1
  Bias/1 -> Pos/1  "Pos Right"
  Bias3/1 -> Vel/1  "Vel Right"
  Bias2/1 -> Mz/1  "Mz Right"
  Bias1/1 -> My/1  "My Right"

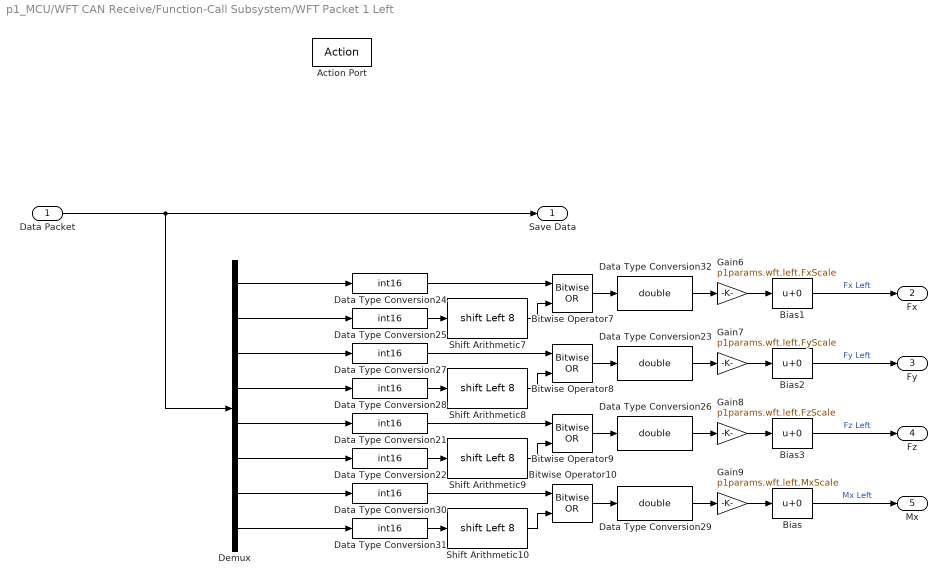
== system p1_MCU/WFT CAN Receive/Function-Call Subsystem/WFT Packet 1 Left ==
  Data Packet : Inport
  Action Port : ActionPort  ActionPortLabel=case [ 460 ]:
  Bias{,1..3} (4 alike) : Bias  SaturateOnIntegerOverflow=off
  Bitwise Operator{7..10} (4 alike) : simulink/Logic and Bit Operations/Bitwise Operator  logicop=OR  UseBitMask=off  NumInputPorts=2  BitMask=bin2dec('11011001')  BitMaskRealWorld=Stored Integer
  Data Type Conversion{21..22,24..25,27..28,30..31} (8 alike) : DataTypeConversion  OutDataTypeStr=int16  SaturateOnIntegerOverflow=off  RndMeth=Floor
  Data Type Conversion{23,26,29,32} (4 alike) : DataTypeConversion  OutDataTypeStr=double  SaturateOnIntegerOverflow=off  RndMeth=Floor
  Demux : Demux  Outputs=8
  Gain6 : Gain  Gain=p1params.wft.left.FxScale  OutDataTypeStr=Inherit: Inherit via back propagation
  Gain7 : Gain  Gain=p1params.wft.left.FyScale  OutDataTypeStr=Inherit: Inherit via back propagation
  Gain8 : Gain  Gain=p1params.wft.left.FzScale  OutDataTypeStr=Inherit: Inherit via back propagation
  Gain9 : Gain  Gain=p1params.wft.left.MxScale  OutDataTypeStr=Inherit: Inherit via back propagation
  Shift Arithmetic{7..10} (4 alike) : ArithShift  BitShiftNumber=8  BitShiftDirection=Left
  Save Data : Outport
  Fx : Outport  Port=2
  Fy : Outport  Port=3
  Fz : Outport  Port=4
  Mx : Outport  Port=5
  wires:
  Data Packet/1 -> Save Data/1, Demux/1
  Demux/8 -> Data Type Conversion31/1
  Demux/7 -> Data Type Conversion30/1
  Demux/6 -> Data Type Conversion22/1
  Demux/5 -> Data Type Conversion21/1
  Demux/4 -> Data Type Conversion28/1
  Demux/3 -> Data Type Conversion27/1
  Demux/2 -> Data Type Conversion25/1
  Demux/1 -> Data Type Conversion24/1
  Data Type Conversion23/1 -> Gain7/1
  Shift Arithmetic9/1 -> Bitwise Operator9/2
  Shift Arithmetic8/1 -> Bitwise Operator8/2
  Data Type Conversion25/1 -> Shift Arithmetic7/1
  Data Type Conversion31/1 -> Shift Arithmetic10/1
  Bitwise Operator7/1 -> Data Type Conversion32/1
  Data Type Conversion29/1 -> Gain9/1
  Data Type Conversion27/1 -> Bitwise Operator8/1
  Shift Arithmetic10/1 -> Bitwise Operator10/2
  Gain6/1 -> Bias1/1
  Bitwise Operator8/1 -> Data Type Conversion23/1
  Bitwise Operator10/1 -> Data Type Conversion29/1
  Data Type Conversion26/1 -> Gain8/1
  Gain8/1 -> Bias3/1
  Shift Arithmetic7/1 -> Bitwise Operator7/2
  Data Type Conversion32/1 -> Gain6/1
  Data Type Conversion28/1 -> Shift Arithmetic8/1
  Gain9/1 -> Bias/1
  Bitwise Operator9/1 -> Data Type Conversion26/1
  Data Type Conversion21/1 -> Bitwise Operator9/1
  Data Type Conversion22/1 -> Shift Arithmetic9/1
  Data Type Conversion30/1 -> Bitwise Operator10/1
  Gain7/1 -> Bias2/1
  Data Type Conversion24/1 -> Bitwise Operator7/1
  Bias/1 -> Mx/1  "Mx Left"
  Bias3/1 -> Fz/1  "Fz Left"
  Bias2/1 -> Fy/1  "Fy Left"
  Bias1/1 -> Fx/1  "Fx Left"

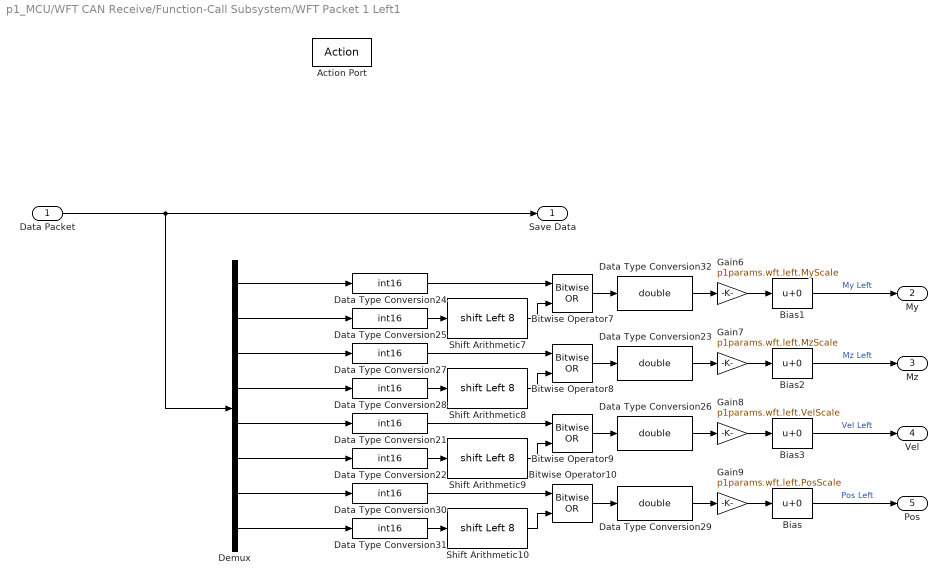
== system p1_MCU/WFT CAN Receive/Function-Call Subsystem/WFT Packet 1 Left1 ==
  Data Packet : Inport
  Action Port : ActionPort  ActionPortLabel=case [ 1484 ]:
  Bias{,1..3} (4 alike) : Bias  SaturateOnIntegerOverflow=off
  Bitwise Operator{7..10} (4 alike) : simulink/Logic and Bit Operations/Bitwise Operator  logicop=OR  UseBitMask=off  NumInputPorts=2  BitMask=bin2dec('11011001')  BitMaskRealWorld=Stored Integer
  Data Type Conversion{21..22,24..25,27..28,30..31} (8 alike) : DataTypeConversion  OutDataTypeStr=int16  SaturateOnIntegerOverflow=off  RndMeth=Floor
  Data Type Conversion{23,26,29,32} (4 alike) : DataTypeConversion  OutDataTypeStr=double  SaturateOnIntegerOverflow=off  RndMeth=Floor
  Demux : Demux  Outputs=8
  Gain6 : Gain  Gain=p1params.wft.left.MyScale  OutDataTypeStr=Inherit: Inherit via back propagation
  Gain7 : Gain  Gain=p1params.wft.left.MzScale  OutDataTypeStr=Inherit: Inherit via back propagation
  Gain8 : Gain  Gain=p1params.wft.left.VelScale  OutDataTypeStr=Inherit: Inherit via back propagation
  Gain9 : Gain  Gain=p1params.wft.left.PosScale  OutDataTypeStr=Inherit: Inherit via back propagation
  Shift Arithmetic{7..10} (4 alike) : ArithShift  BitShiftNumber=8  BitShiftDirection=Left
  Save Data : Outport
  My : Outport  Port=2
  Mz : Outport  Port=3
  Vel : Outport  Port=4
  Pos : Outport  Port=5
  wires:
  Data Packet/1 -> Save Data/1, Demux/1
  Demux/8 -> Data Type Conversion31/1
  Demux/7 -> Data Type Conversion30/1
  Demux/6 -> Data Type Conversion22/1
  Demux/5 -> Data Type Conversion21/1
  Demux/4 -> Data Type Conversion28/1
  Demux/3 -> Data Type Conversion27/1
  Demux/2 -> Data Type Conversion25/1
  Demux/1 -> Data Type Conversion24/1
  Data Type Conversion23/1 -> Gain7/1
  Shift Arithmetic9/1 -> Bitwise Operator9/2
  Shift Arithmetic8/1 -> Bitwise Operator8/2
  Data Type Conversion25/1 -> Shift Arithmetic7/1
  Data Type Conversion31/1 -> Shift Arithmetic10/1
  Bitwise Operator7/1 -> Data Type Conversion32/1
  Data Type Conversion29/1 -> Gain9/1
  Data Type Conversion27/1 -> Bitwise Operator8/1
  Shift Arithmetic10/1 -> Bitwise Operator10/2
  Gain6/1 -> Bias1/1
  Bitwise Operator8/1 -> Data Type Conversion23/1
  Bitwise Operator10/1 -> Data Type Conversion29/1
  Data Type Conversion26/1 -> Gain8/1
  Gain8/1 -> Bias3/1
  Shift Arithmetic7/1 -> Bitwise Operator7/2
  Data Type Conversion32/1 -> Gain6/1
  Data Type Conversion28/1 -> Shift Arithmetic8/1
  Gain9/1 -> Bias/1
  Bitwise Operator9/1 -> Data Type Conversion26/1
  Data Type Conversion21/1 -> Bitwise Operator9/1
  Data Type Conversion22/1 -> Shift Arithmetic9/1
  Data Type Conversion30/1 -> Bitwise Operator10/1
  Gain7/1 -> Bias2/1
  Data Type Conversion24/1 -> Bitwise Operator7/1
  Bias/1 -> Pos/1  "Pos Left"
  Bias3/1 -> Vel/1  "Vel Left"
  Bias2/1 -> Mz/1  "Mz Left"
  Bias1/1 -> My/1  "My Left"

== system p1_MCU/WFT CAN Receive/Function-Call Subsystem/WFT Packet 1 Left2 ==
  Data Packet : Inport
  Action Port : ActionPort  ActionPortLabel=case [ 972 ]:
  Bias1 : Bias  SaturateOnIntegerOverflow=off
  Bias2 : Bias  SaturateOnIntegerOverflow=off
  Bitwise Operator7 : simulink/Logic and Bit Operations/Bitwise Operator  logicop=OR  UseBitMask=off  NumInputPorts=2  BitMask=bin2dec('11011001')  BitMaskRealWorld=Stored Integer
  Bitwise Operator8 : simulink/Logic and Bit Operations/Bitwise Operator  logicop=OR  UseBitMask=off  NumInputPorts=2  BitMask=bin2dec('11011001')  BitMaskRealWorld=Stored Integer
  Data Type Conversion23 : DataTypeConversion  OutDataTypeStr=double  SaturateOnIntegerOverflow=off  RndMeth=Floor
  Data Type Conversion{24..25,27..28} (4 alike) : DataTypeConversion  OutDataTypeStr=int16  SaturateOnIntegerOverflow=off  RndMeth=Floor
  Data Type Conversion32 : DataTypeConversion  OutDataTypeStr=double  SaturateOnIntegerOverflow=off  RndMeth=Floor
  Demux : Demux
  Gain6 : Gain  Gain=p1params.wft.left.AxScale  OutDataTypeStr=Inherit: Inherit via back propagation
  Gain7 : Gain  Gain=p1params.wft.left.AzScale  OutDataTypeStr=Inherit: Inherit via back propagation
  Selector : Selector  InputPortWidth=8  IndexOptions=Index vector (dialog)  Indices=[1:4]  OutputSizes=1
  Shift Arithmetic7 : ArithShift  BitShiftNumber=8  BitShiftDirection=Left
  Shift Arithmetic8 : ArithShift  BitShiftNumber=8  BitShiftDirection=Left
  Save Data : Outport
  Ax : Outport  Port=2
  Az : Outport  Port=3
  wires:
  Data Packet/1 -> Selector/1, Demux/1
  Demux/4 -> Data Type Conversion28/1
  Demux/3 -> Data Type Conversion27/1
  Demux/2 -> Data Type Conversion25/1
  Demux/1 -> Data Type Conversion24/1
  Data Type Conversion23/1 -> Gain7/1
  Shift Arithmetic8/1 -> Bitwise Operator8/2
  Data Type Conversion25/1 -> Shift Arithmetic7/1
  Bitwise Operator7/1 -> Data Type Conversion32/1
  Data Type Conversion27/1 -> Bitwise Operator8/1
  Gain6/1 -> Bias1/1
  Bitwise Operator8/1 -> Data Type Conversion23/1
  Shift Arithmetic7/1 -> Bitwise Operator7/2
  Data Type Conversion32/1 -> Gain6/1
  Data Type Conversion28/1 -> Shift Arithmetic8/1
  Gain7/1 -> Bias2/1
  Data Type Conversion24/1 -> Bitwise Operator7/1
  Bias2/1 -> Az/1  "Az Left"
  Bias1/1 -> Ax/1  "Ax Left"
  Selector/1 -> Save Data/1

== system p1_MCU/WFT CAN Receive/Function-Call Subsystem/WFT Packet 1 Left3 ==
  Data Packet : Inport
  Action Port : ActionPort  ActionPortLabel=case [ 967 ]:
  Bias1 : Bias  SaturateOnIntegerOverflow=off
  Bias2 : Bias  SaturateOnIntegerOverflow=off
  Bitwise Operator7 : simulink/Logic and Bit Operations/Bitwise Operator  logicop=OR  UseBitMask=off  NumInputPorts=2  BitMask=bin2dec('11011001')  BitMaskRealWorld=Stored Integer
  Bitwise Operator8 : simulink/Logic and Bit Operations/Bitwise Operator  logicop=OR  UseBitMask=off  NumInputPorts=2  BitMask=bin2dec('11011001')  BitMaskRealWorld=Stored Integer
  Data Type Conversion23 : DataTypeConversion  OutDataTypeStr=double  SaturateOnIntegerOverflow=off  RndMeth=Floor
  Data Type Conversion{24..25,27..28} (4 alike) : DataTypeConversion  OutDataTypeStr=int16  SaturateOnIntegerOverflow=off  RndMeth=Floor
  Data Type Conversion32 : DataTypeConversion  OutDataTypeStr=double  SaturateOnIntegerOverflow=off  RndMeth=Floor
  Demux : Demux
  Gain6 : Gain  Gain=p1params.wft.right.AxScale  OutDataTypeStr=Inherit: Inherit via back propagation
  Gain7 : Gain  Gain=p1params.wft.right.AzScale  OutDataTypeStr=Inherit: Inherit via back propagation
  Selector : Selector  InputPortWidth=8  IndexOptions=Index vector (dialog)  Indices=[1:4]  OutputSizes=1
  Shift Arithmetic7 : ArithShift  BitShiftNumber=8  BitShiftDirection=Left
  Shift Arithmetic8 : ArithShift  BitShiftNumber=8  BitShiftDirection=Left
  Save Data : Outport
  Ax : Outport  Port=2
  Az : Outport  Port=3
  wires:
  Bias1/1 -> Ax/1  "Ax Right"
  Bias2/1 -> Az/1  "Az RIght"
  Data Type Conversion24/1 -> Bitwise Operator7/1
  Gain7/1 -> Bias2/1
  Data Type Conversion28/1 -> Shift Arithmetic8/1
  Data Type Conversion32/1 -> Gain6/1
  Shift Arithmetic7/1 -> Bitwise Operator7/2
  Bitwise Operator8/1 -> Data Type Conversion23/1
  Gain6/1 -> Bias1/1
  Data Type Conversion27/1 -> Bitwise Operator8/1
  Bitwise Operator7/1 -> Data Type Conversion32/1
  Data Type Conversion25/1 -> Shift Arithmetic7/1
  Shift Arithmetic8/1 -> Bitwise Operator8/2
  Data Type Conversion23/1 -> Gain7/1
  Demux/1 -> Data Type Conversion24/1
  Demux/2 -> Data Type Conversion25/1
  Demux/3 -> Data Type Conversion27/1
  Demux/4 -> Data Type Conversion28/1
  Data Packet/1 -> Demux/1, Selector/1
  Selector/1 -> Save Data/1

== system p1_MCU/Steering Control/Steering Controller/HAL-9000/Chirp Signal ==
  note: freqSlope = deltaFreq/targetTime;
      | instantaneousFreq(t) = freqSlope*t + initialFreq;
      | intantaneousPhase(t) = integral(instFreq) = ...
      |       0.5*freqSlope*t^2 + initialFreq*t;
      | outputSignal(t) = sin(instantaneousPhase(t));
  Start Time : Inport
  Digital Clock : DigitalClock  SampleTime=Ts_MCU
  Gain : Gain  DisableCoverage=on  Gain=0.5  OutDataTypeStr=Inherit: Same as input  ParamDataTypeStr=Inherit: Same as input
  Output : Trigonometry
  Product : Product  DisableCoverage=on  Inputs=*/  InputSameDT=on  SaturateOnIntegerOverflow=on  OutDataTypeStr=Inherit: Same as first input
  Product1 : Product  DisableCoverage=on  InputSameDT=on  SaturateOnIntegerOverflow=on  OutDataTypeStr=Inherit: Same as first input
  Product2 : Product  DisableCoverage=on  InputSameDT=on  SaturateOnIntegerOverflow=on  OutDataTypeStr=Inherit: Same as first input
  Saturation : Saturate  UpperLimit=duration  LowerLimit=0
  Sum : Sum  DisableCoverage=on  Inputs=|++  InputSameDT=on  SaturateOnIntegerOverflow=on  OutDataTypeStr=Inherit: Same as first input
  Sum1 : Sum  DisableCoverage=on  Inputs=-+|  InputSameDT=on  SaturateOnIntegerOverflow=on  OutDataTypeStr=Inherit: Same as first input
  deltaFreq : Constant  DisableCoverage=on  Value=2*pi*(f2-f1)
  initialFreq : Constant  DisableCoverage=on  Value=2*pi*f1
  targetTime : Constant  DisableCoverage=on  Value=T
  Out2 : Outport
  wires:
  Sum1/1 -> Saturation/1
  Digital Clock/1 -> Sum1/2
  Start Time/1 -> Sum1/1
  deltaFreq/1 -> Product/1
  targetTime/1 -> Product/2
  Product/1 -> Gain/1
  Gain/1 -> Product1/2
  Product1/1 -> Sum/1
  initialFreq/1 -> Sum/2
  Sum/1 -> Product2/2
  Product2/1 -> Output/1
  Output/1 -> Out2/1
  Saturation/1 -> Product1/1, Product2/1

== system p1_MCU/Steering Control/Steering Controller/HAL-9000/Double chirp ==
  In1 : Inport
  Chirp One : Subsystem  mask(chirp){f1=startfreq, T=duration/2, f2=endfreq, VectorParams1D=on}
      mask prompts: f1 "Initial frequency (Hz):"; T "Target time (secs):"; f2 "Frequency at target time (Hz):"; VectorParams1D "Interpret vectors parameters as 1-D"
      mask help: Output a linear chirp signal (sine wave whose frequency varies linearly with time).
      mask init: same as p1_MCU/Steering Control/Steering Controller/HAL-9000/Chirp Signal
      mask Help: The chirp signal has linearly increasing frequency with time.  This block can be used for spectral analysis of nonlinear systems.
      mask Display: plot(t,sin(t.*t))
  Chirp Two : Subsystem  mask(chirp){f1=startfreq, T=duration/2, f2=endfreq, VectorParams1D=on}
      mask prompts: f1 "Initial frequency (Hz):"; T "Target time (secs):"; f2 "Frequency at target time (Hz):"; VectorParams1D "Interpret vectors parameters as 1-D"
      mask help: Output a linear chirp signal (sine wave whose frequency varies linearly with time).
      mask init: same as p1_MCU/Steering Control/Steering Controller/HAL-9000/Chirp Signal
      mask Help: The chirp signal has linearly increasing frequency with time.  This block can be used for spectral analysis of nonlinear systems.
      mask Display: plot(t,sin(t.*t))
  Digital Clock : DigitalClock  SampleTime=Ts_MCU
  Relational Operator : RelationalOperator  Operator=<=  OutDataTypeStr=float('double')  InputSameDT=off
  Sum : Sum  DisableCoverage=on  Inputs=++|  InputSameDT=on  SaturateOnIntegerOverflow=on  OutDataTypeStr=Inherit: Same as first input
  Switch : Switch  Threshold=.5  SaturateOnIntegerOverflow=off  InputSameDT=off
  initialFreq : Constant  DisableCoverage=on  Value=duration/2
  Out1 : Outport
  wires:
  Digital Clock/1 -> Relational Operator/1
  Relational Operator/1 -> Switch/2
  initialFreq/1 -> Sum/2
  Sum/1 -> Relational Operator/2, Chirp Two/1(Start Time)
  In1/1 -> Sum/1, Chirp One/1(Start Time)
  Switch/1 -> Out1/1
  Chirp Two/1(Out2) -> Switch/3
  Chirp One/1(Out2) -> Switch/1

== system p1_MCU/Steering Control/Steering Controller/HAL-9000/Double-step ==
  Start Time : Inport
  Data Type Conversion : DataTypeConversion  OutDataTypeStr=double  SaturateOnIntegerOverflow=off  RndMeth=Floor
  Data Type Conversion1 : DataTypeConversion  OutDataTypeStr=double  SaturateOnIntegerOverflow=off  RndMeth=Floor
  Digital Clock : DigitalClock  SampleTime=Ts_MCU
  Left Pulse : simulink/Logic and Bit Operations/Interval Test  IntervalClosedRight=off  uplimit=duration  IntervalClosedLeft=on  lowlimit=0  OutDataTypeStr=boolean
  Right Pulse : simulink/Logic and Bit Operations/Interval Test  IntervalClosedRight=off  uplimit=3*duration  IntervalClosedLeft=on  lowlimit=2*duration  OutDataTypeStr=boolean
  Sum : Sum  Inputs=+|-
  Sum1 : Sum  Inputs=+|-
  Out : Outport
  wires:
  Data Type Conversion1/1 -> Sum1/2
  Data Type Conversion/1 -> Sum1/1
  Left Pulse/1 -> Data Type Conversion/1
  Right Pulse/1 -> Data Type Conversion1/1
  Sum1/1 -> Out/1
  Sum/1 -> Right Pulse/1, Left Pulse/1
  Digital Clock/1 -> Sum/1
  Start Time/1 -> Sum/2
